simulink model "lqr_controller"  (R2018b)
settings: Solver=VariableStepAuto  StartTime=0.0  StopTime=10.0  RelTol=1e-3
values from neighbouring files (symbols this model uses):
  A = [0 1 0 0 ... (first row only)    [kalman.m]    (also in lqr_controller.m; lqr_observare.m; state_space.m)
  B = [0 ... (first row only)    [kalman.m]    (also in lqr_controller.m; lqr_observare.m; state_space.m)
  C = [1 0 0 0;]    [kalman.m]    (also in lqr_controller.m = [1 0 0 0; lqr_observare.m = [1 0 0 0; state_space.m = [1 0 0 0)
  K = lqr(A,B,Q,R)    [lqr_controller.m]    (also in state_space.m = eig(A))
settings Model: Creator=SAFARBALI  LastModifiedBy=888
settings SFSimCC: SimUseLocalCustomCode=off
settings RTWCC: RTWUseLocalCustomCode=off
settings CodeAppCC: StateflowObjectComments=on

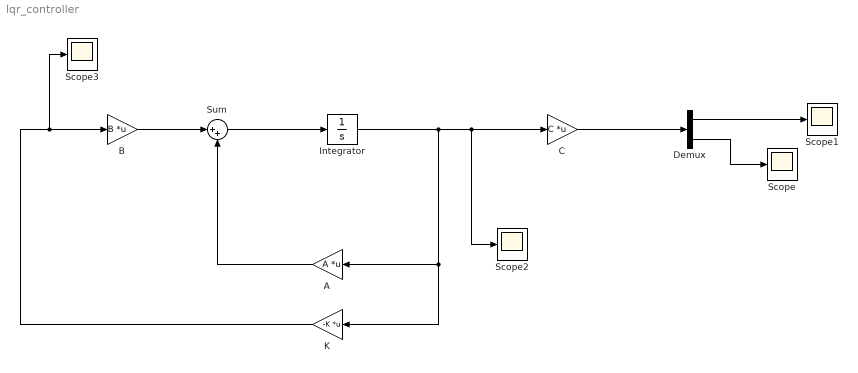
== system lqr_controller ==
  A : Gain  Gain=A  Multiplication=Matrix(K*u)
  B : Gain  Gain=B  Multiplication=Matrix(K*u)
  C : Gain  Gain=C  Multiplication=Matrix(K*u)
  Demux : Demux  Outputs=2
  Integrator : Integrator  InitialCondition=[0;5;0;0]
  K : Gain  Gain=-K  Multiplication=Matrix(K*u)
  Scope{,1..3} (4 alike) : Scope
  Sum : Sum  Inputs=|++
  wires:
  Integrator/1 -> K/1, A/1, Scope2/1, C/1
  Sum/1 -> Integrator/1
  B/1 -> Sum/1
  A/1 -> Sum/2
  K/1 -> Scope3/1, B/1
  C/1 -> Demux/1
  Demux/1 -> Scope1/1
  Demux/2 -> Scope/1
